simulink model "thrust_allocation"  (R2020a)
settings: Solver=FixedStepAuto  StartTime=0.0  StopTime=10.0  FixedStep=0.01  RelTol=1e-3
PreLoadFcn:
  | load("interfaces.mat");
libraries: simulink_extras x4
settings Model: Creator=thomas.evang  LastModifiedBy=thomas.evang
settings SFSimCC: CustomCodeUndefinedFunction=UseInterfaceOnly
settings RTWCC: Description=Generic Real-Time Target  RetainRTWFile=on

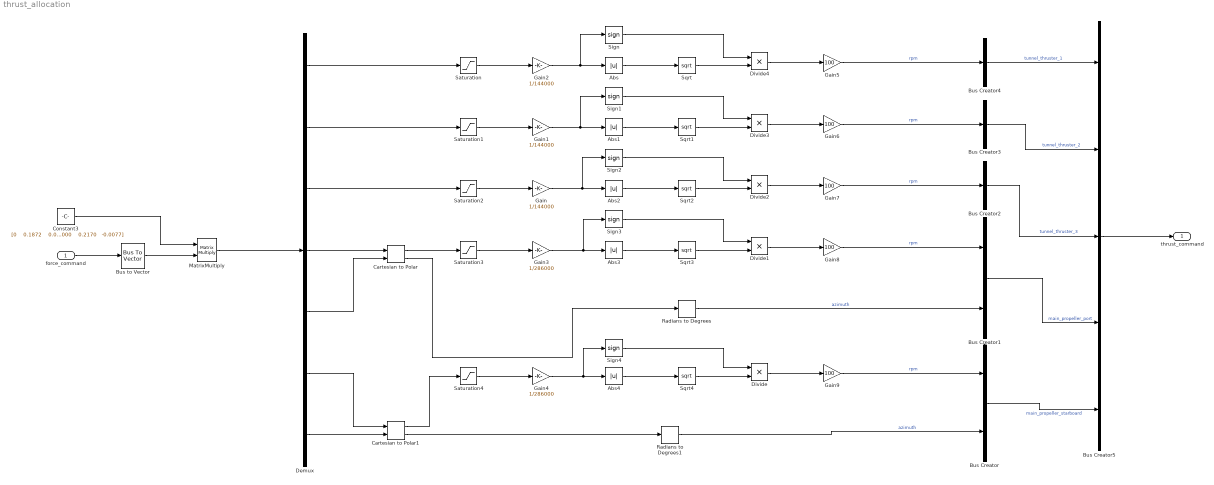
== system thrust_allocation ==
  force_command : Inport  OutDataTypeStr=Bus: force_3dof
  Abs{,1..4} (5 alike) : Abs
  Bus Creator : BusCreator  Inputs=2  OutDataTypeStr=Bus: azimuth_thruster_command
      settings: InheritFromInputs=off
  Bus Creator1 : BusCreator  Inputs=2  OutDataTypeStr=Bus: azimuth_thruster_command
      settings: InheritFromInputs=off
  Bus Creator2 : BusCreator  Inputs=1  OutDataTypeStr=Bus: tunnel_thruster_command
      settings: InheritFromInputs=off
  Bus Creator3 : BusCreator  Inputs=1  OutDataTypeStr=Bus: tunnel_thruster_command
      settings: InheritFromInputs=off
  Bus Creator4 : BusCreator  Inputs=1  OutDataTypeStr=Bus: tunnel_thruster_command
      settings: InheritFromInputs=off
  Bus Creator5 : BusCreator  Inputs=5  OutDataTypeStr=Bus: thrust_command
      settings: InheritFromInputs=off
  Bus to Vector : BusToVector
  Cartesian to Polar : simulink_extras/Transformations/Cartesian to Polar
  Cartesian to Polar1 : simulink_extras/Transformations/Cartesian to Polar
  Constant3 : Constant  Value=|
      | [0    0.1872    0.0058;
      |     0.0000    0.1886    0.0051;
      |     0.0000    0.1901    0.0045;
      |     0.5000   -0.0018    0.0008;
      |     0.0000    0.2170   -0.0077;
      |     0.5000    0.0018   -0.0008;
      |     0.0000    0.2170   -0.0077]
  Demux : Demux  Outputs=7
  Divide{,1..4} (5 alike) : Product
  Gain : Gain  Gain=1/144000
  Gain1 : Gain  Gain=1/144000
  Gain2 : Gain  Gain=1/144000
  Gain3 : Gain  Gain=1/286000
  Gain4 : Gain  Gain=1/286000
  Gain{5..9} (5 alike) : Gain  Gain=100
  MatrixMultiply : Product  Multiplication=Matrix(*)
  Radians to Degrees : simulink_extras/Transformations/Radians to Degrees
  Radians to Degrees1 : simulink_extras/Transformations/Radians to Degrees
  Saturation : Saturate  UpperLimit=144000  LowerLimit=-144000
  Saturation1 : Saturate  UpperLimit=144000  LowerLimit=-144000
  Saturation2 : Saturate  UpperLimit=144000  LowerLimit=-144000
  Saturation3 : Saturate  UpperLimit=286000  LowerLimit=0
  Saturation4 : Saturate  UpperLimit=286000  LowerLimit=0
  Sign{,1..4} (5 alike) : Signum
  Sqrt{,1..4} (5 alike) : Sqrt  SaturateOnIntegerOverflow=on
  thrust_command : Outport  OutDataTypeStr=Bus: thrust_command  VectorParamsAs1DForOutWhenUnconnected=off
  wires:
  Demux/7 -> Cartesian to Polar1/2
  Sign/1 -> Divide4/1
  Gain6/1 -> Bus Creator3/1  "rpm"
  Gain5/1 -> Bus Creator4/1  "rpm"
  Gain7/1 -> Bus Creator2/1  "rpm"
  Abs/1 -> Sqrt/1
  Divide3/1 -> Gain6/1
  Gain3/1 -> Sign3/1, Abs3/1
  Gain4/1 -> Sign4/1, Abs4/1
  Radians to Degrees1/1 -> Bus Creator/2  "azimuth"
  Demux/5 -> Cartesian to Polar/2
  Sqrt3/1 -> Divide1/2
  Radians to Degrees/1 -> Bus Creator1/2  "azimuth"
  Divide4/1 -> Gain5/1
  Divide2/1 -> Gain7/1
  Demux/2 -> Saturation1/1
  Saturation4/1 -> Gain4/1
  Cartesian to Polar1/1 -> Saturation4/1
  Sign3/1 -> Divide1/1
  Sign4/1 -> Divide/1
  Demux/6 -> Cartesian to Polar1/1
  Demux/4 -> Cartesian to Polar/1
  Sign1/1 -> Divide3/1
  Demux/1 -> Saturation/1
  Demux/3 -> Saturation2/1
  Saturation/1 -> Gain2/1
  Sqrt2/1 -> Divide2/2
  Sqrt1/1 -> Divide3/2
  Abs4/1 -> Sqrt4/1
  MatrixMultiply/1 -> Demux/1
  Saturation2/1 -> Gain/1
  Gain/1 -> Sign2/1, Abs2/1
  Abs3/1 -> Sqrt3/1
  Abs1/1 -> Sqrt1/1
  Divide/1 -> Gain9/1
  Cartesian to Polar/1 -> Saturation3/1
  Gain8/1 -> Bus Creator1/1  "rpm"
  Saturation3/1 -> Gain3/1
  Saturation1/1 -> Gain1/1
  Sqrt/1 -> Divide4/2
  Constant3/1 -> MatrixMultiply/1
  Sqrt4/1 -> Divide/2
  Gain1/1 -> Sign1/1, Abs1/1
  Sign2/1 -> Divide2/1
  force_command/1 -> Bus to Vector/1
  Gain2/1 -> Sign/1, Abs/1
  Abs2/1 -> Sqrt2/1
  Divide1/1 -> Gain8/1
  Bus to Vector/1 -> MatrixMultiply/2
  Gain9/1 -> Bus Creator/1  "rpm"
  Bus Creator1/1 -> Bus Creator5/4  "main_propeller_port"
  Bus Creator/1 -> Bus Creator5/5  "main_propeller_starboard"
  Bus Creator2/1 -> Bus Creator5/3  "tunnel_thruster_3"
  Bus Creator3/1 -> Bus Creator5/2  "tunnel_thruster_2"
  Bus Creator4/1 -> Bus Creator5/1  "tunnel_thruster_1"
  Bus Creator5/1 -> thrust_command/1
  Cartesian to Polar1/2 -> Radians to Degrees1/1
  Cartesian to Polar/2 -> Radians to Degrees/1
